simulink model "ILC"  (R2021a)
settings: Solver=VariableStepAuto  StartTime=0.0  StopTime=5  RelTol=1e-3
libraries: robotmaniplib x1, robotcorelib x1
settings Model: Creator=ASUS  LastModifiedBy=ASUS

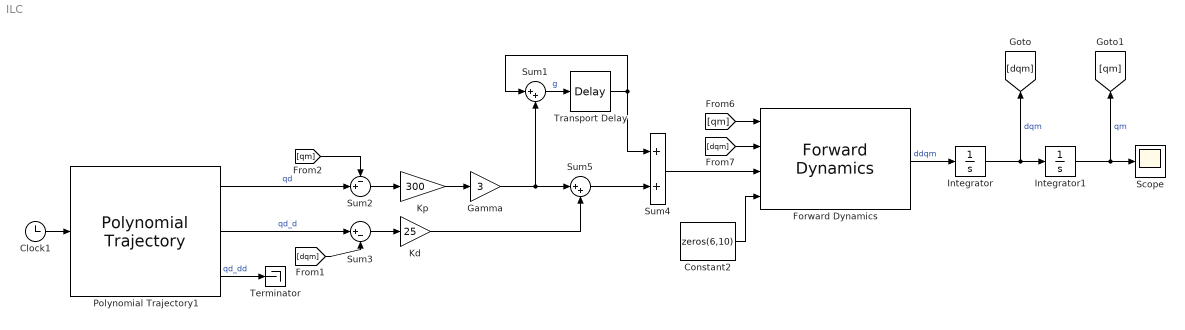
== system ILC ==
  Clock1 : Clock
  Constant2 : Constant  Value=zeros(6,10)
  Forward Dynamics : robotmaniplib/Forward Dynamics  RigidBodyTree=robot  SimulateUsing=Code generation
  Gamma : Gain  Gain=3
  Integrator : Integrator
  Integrator1 : Integrator
  Kd : Gain  Gain=25
  Kp : Gain  Gain=300
  Polynomial Trajectory1 : robotcorelib/Polynomial Trajectory  WaypointSource=Internal  Waypoints=[ pi/4 pi/4; pi/2 pi/2; pi/8 pi/8; pi/3 pi/3; pi/4 pi/4; pi/5 pi/5]  TimePoints=[ 0, 0.01 ]  TimeInterval=[ 1, 4 ]  Method=Cubic Polynomial  ParameterSource=Internal  VelocityBoundaryCondition=zeros( 6, 2 )  AccelerationBoundaryCondition=zeros( 2, 5 )  SimulateUsing=Interpreted execution
  Scope : Scope
  Sum1 : Sum  Inputs=|++
  Sum2 : Sum  Inputs=-+|
  Sum3 : Sum  Inputs=|+-
  Sum4 : Sum
  Sum5 : Sum  Inputs=|++
  Terminator : Terminator
  Transport Delay : TransportDelay  DelayTime=2.5
  wires:
  Forward Dynamics/1 -> Integrator/1  "ddqm"
  Integrator/1 -> [dqm], Integrator1/1  "dqm"
  Constant2/1 -> Forward Dynamics/4
  Integrator1/1 -> [qm], Scope/1  "qm"
  [qm] -> Forward Dynamics/1
  [dqm] -> Forward Dynamics/2
  [qm] -> Sum2/1
  Clock1/1 -> Polynomial Trajectory1/1
  Polynomial Trajectory1/1 -> Sum2/2  "qd"
  [dqm] -> Sum3/2
  Sum2/1 -> Kp/1
  Kp/1 -> Gamma/1
  Polynomial Trajectory1/2 -> Sum3/1  "qd_d"
  Sum3/1 -> Kd/1
  Kd/1 -> Sum5/2
  Gamma/1 -> Sum1/2, Sum5/1
  Polynomial Trajectory1/3 -> Terminator/1  "qd_dd"
  Sum5/1 -> Sum4/2
  Sum4/1 -> Forward Dynamics/3
  Sum1/1 -> Transport Delay/1  "g"
  Transport Delay/1 -> Sum4/1, Sum1/1
